simulink model "N_scheme_S5"  (R2024b)
settings: Solver=VariableStepAuto  StartTime=0.0  StopTime=10.0  RelTol=1e-3
values from neighbouring files (symbols this model uses):
  Ga = 0.095    [lab09_01_01.m]
  Gf = 1    [lab09_01_01.m]
  Gs = 1    [lab09_01_01.m]
  Kn = (K_max+K_min)/2    (= 12.5)    [lab09_01_01.m]
  p1_n = (p1_min + p1_max)/2    (= 0.8)    [lab09_01_01.m]
  p2_n = (p2_min + p2_max)/2    (= 2.5)    [lab09_01_01.m]
  wk = (K_max-K_min)/2    (= 5.5)    [lab09_01_01.m]
  wp1 = (p1_max- p1_min)/2    (= 0.35)    [lab09_01_01.m]
  wp2 = (p2_max - p2_min)/2    (= 1)    [lab09_01_01.m]
libraries: cstblocks x2
settings Model: Creator=adrian  LastModifiedBy=adrian

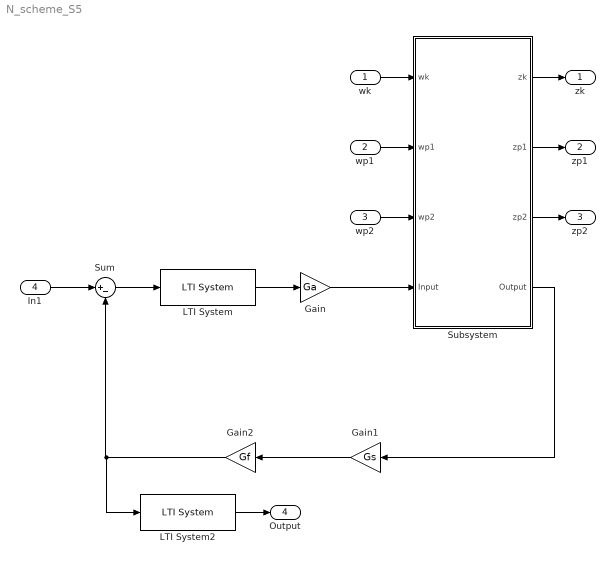
== system N_scheme_S5 ==
  wk : Inport
  wp1 : Inport  Port=2
  wp2 : Inport  Port=3
  In1 : Inport  Port=4
  Gain : Gain  Gain=Ga
  Gain1 : Gain  Gain=Gs
  Gain2 : Gain  Gain=Gf
  LTI System : cstblocks/LTI System  sys=Gc  IC=[]  PadeOrder=0
  LTI System2 : cstblocks/LTI System  sys=WT_mu_s5  IC=[]  PadeOrder=0
  Subsystem : Subsystem
  Sum : Sum  Inputs=|+-
  zk : Outport
  zp1 : Outport  Port=2
  zp2 : Outport  Port=3
  Output : Outport  Port=4
  wires:
  Gain/1 -> Subsystem/4(Input)
  LTI System/1 -> Gain/1
  Gain1/1 -> Gain2/1
  Subsystem/4(Output) -> Gain1/1
  Sum/1 -> LTI System/1
  wk/1 -> Subsystem/1(wk)
  wp1/1 -> Subsystem/2(wp1)
  wp2/1 -> Subsystem/3(wp2)
  Subsystem/1(zk) -> zk/1
  Subsystem/2(zp1) -> zp1/1
  Subsystem/3(zp2) -> zp2/1
  In1/1 -> Sum/1
  Gain2/1 -> LTI System2/1, Sum/2
  LTI System2/1 -> Output/1

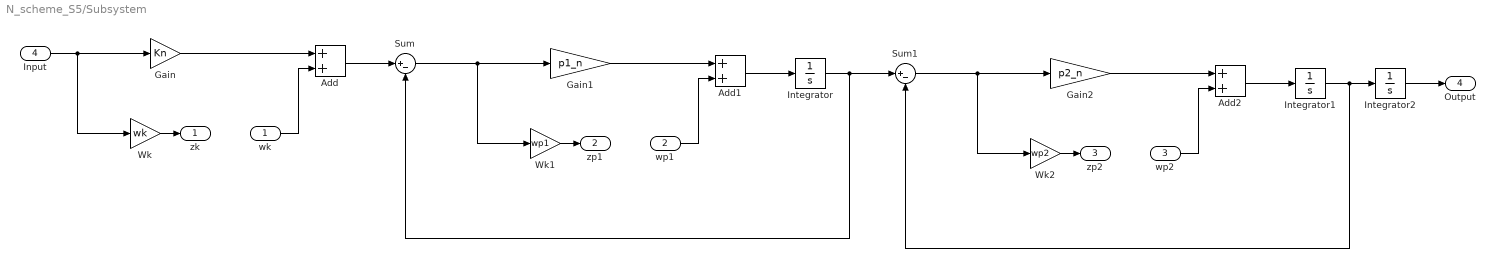
== system N_scheme_S5/Subsystem ==
  wk : Inport
  wp1 : Inport  Port=2
  wp2 : Inport  Port=3
  Input : Inport  Port=4
  Add : Sum
  Add1 : Sum
  Add2 : Sum
  Gain : Gain  Gain=Kn
  Gain1 : Gain  Gain=p1_n
  Gain2 : Gain  Gain=p2_n
  Integrator : Integrator
  Integrator1 : Integrator
  Integrator2 : Integrator
  Sum : Sum  Inputs=|+-
  Sum1 : Sum  Inputs=|+-
  Wk : Gain  Gain=wk
  Wk1 : Gain  Gain=wp1
  Wk2 : Gain  Gain=wp2
  zk : Outport
  zp1 : Outport  Port=2
  zp2 : Outport  Port=3
  Output : Outport  Port=4
  wires:
  Input/1 -> Wk/1, Gain/1
  Wk/1 -> zk/1
  Gain/1 -> Add/1
  wk/1 -> Add/2
  Wk1/1 -> zp1/1
  wp1/1 -> Add1/2
  Gain1/1 -> Add1/1
  Sum/1 -> Wk1/1, Gain1/1
  Add/1 -> Sum/1
  Add1/1 -> Integrator/1
  Integrator1/1 -> Integrator2/1, Sum1/2
  Add2/1 -> Integrator1/1
  Integrator/1 -> Sum1/1, Sum/2
  Sum1/1 -> Gain2/1, Wk2/1
  Gain2/1 -> Add2/1
  wp2/1 -> Add2/2
  Wk2/1 -> zp2/1
  Integrator2/1 -> Output/1
